simulink model "HEV_Simu_V1_1_SfuncPtbs"  (R2018b)
settings: configuration reference "Config_Plant" (kept outside this file)
PreLoadFcn:
  | HevSimuVccWs_V1_PreLoad
  | %プラントモデルのコールバック・プリロード関数のバス定義
  | Driver_PreLoad
  | HEVPlant_Ptbs_V1_BusInfo
  | CtrlStrct_SmplCAN_BusInfo
StartFcn:
  | tic
StopFcn:
  | toc
  | disp(['実時間の' num2str(max(tout)/toc) '倍速'])
libraries: CAN_Lib_V1 x4, simulink x2
settings Model: Creator=E00026  LastModifiedBy=E00026
settings ConfigSetRef: SourceLocation=Base Workspace

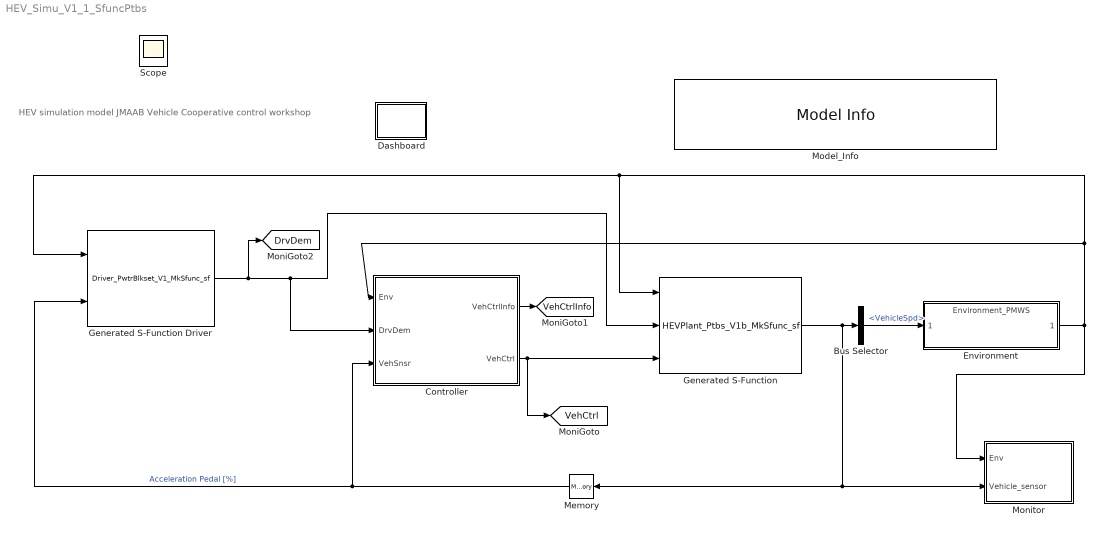
== system HEV_Simu_V1_1_SfuncPtbs ==
  note: HEV simulation model
      | JMAAB Vehicle Cooperative control workshop
  Bus Selector : BusSelector  OutputSignals=Brake_sensor.VehicleSpd
  Controller : Subsystem  TreatAsAtomicUnit=on  VariantControl=VarObj_CtrlStruct_CAN_VNT_Level_2
  Dashboard : Subsystem
  Environment : ModelReference  ModelNameDialog=Environment_PMWS.slx  SimulationMode=Normal  ModelReferenceVersion=1.1287
  Generated S-Function : S-Function  FunctionName=HEVPlant_Ptbs_V1b_MkSfunc_sf  Parameters=sfcnParam1, sfcnParam2, sfcnParam3, sfcnParam4, sfcnParam5, sfcnParam6, sfcnParam7, sfcnParam8, sfcnParam9, sfcnParam10, sfcnParam11, sfcnParam12, sfcnParam13, sfcnParam14, sfcnParam15, sfcnParam16, sfcnParam17, sfcnParam18, sfcnParam19, sfcnParam20, sfcnParam21, sfcnParam22, sfcnParam23, sfcnParam24, sfcnParam25, sfcnParam26, sfcnParam27, sfcnParam28, sfcnParam29, sfcnParam30, sfcnParam31, sfcnParam32, sfcnParam33, sfcnParam34, sfcnParam35, sfcnParam36, sfcnParam37, sfcnParam38, sfcnParam39, sfcnParam40, sfcnParam41, sfcnParam42, sfcnParam43, sfcnParam44, sfcnParam45, sfcnParam46, sfcnParam47, sfcnParam48, sfcnParam49, sfcnParam50, sfcnParam51, sfcnParam52, sfcnParam53, sfcnParam54, sfcnParam55, sfcnParam56, sfcnParam57, sfcnParam58, sfcnParam59, sfcnParam60, sfcnParam61, sfcnParam62, sfcnParam63, sfcnParam64, sfcnParam65, sfcnParam66, sfcnParam67, sfcnParam68, sfcnParam69, sfcnParam70, sfcnParam71, sfcnParam72, sfcnParam73, sfcnParam74, sfcnParam75, sfcnParam76, sfcnParam77, sfcnParam78, sfcnParam79, sfcnParam80, sfcnParam81, sfcnParam82, sfcnParam83, sfcnParam84, sfcnParam85, sfcnParam86, sfcnParam87, sfcnParam88, sfcnParam89, sfcnParam90, sfcnParam91, sfcnParam92, sfcnParam93, sfcnParam94, sfcnParam95, sfcnParam96, sfcnParam97, sfcnParam98, sfcnParam99, sfcnParam100, sfcnParam101, sfcnParam102, sfcnParam103, sfcnParam104, sfcnParam105, sfcnParam106, sfcnParam107, sfcnParam108, sfcnParam109, sfcnParam110, sfcnParam111, sfcnParam112, sfcnParam113, sfcnParam114, sfcnParam115, sfcnParam116, sfcnParam117, sfcnParam118, sfcnParam119, sfcnParam120, sfcnParam121, sfcnParam122, sfcnParam123  SFunctionModules=""  SFunctionDeploymentMode=off  EnableBusSupport=off  mask{rtw_sf_name=HEVPlant_Ptbs_V1b_MkSfunc_sf, showVar=off, sfcnParam1=[3.421], sfcnParam2=[1.0], sfcnParam3=[0.3], sfcnParam4=[10.0], sfcnParam5=[10.0], sfcnParam6=[5000.0], sfcnParam7=[1000.0], sfcnParam8=[0.1], sfcnParam9=[2.27], sfcnParam10=[4.2], sfcnParam11=[7.0], sfcnParam12=[243.1, 253.1, 263.1, 273.1, 283.1, 298.1, 313.1], sfcnParam13=[0.0, 0.01, 0.02, 0.03, 0.04, 0.05, 0.06, 0.07, 0.08, 0.09, 0.1, 0.11, 0.12, 0.13, 0.14, 0.15, 0.16, 0.17, 0.18, 0.19, 0.2, 0.21, 0.22, 0.23, 0.24, 0.25, 0.26, 0.27, 0.28, 0.29, 0.3, 0.31, 0.32, 0.33, 0.34, 0.35, 0.36, 0.37, 0.38, 0.39, 0.4, 0.41, 0.42, 0.43, 0.44, 0.45, 0.46, 0.47, 0.48, 0.49, 0.5, 0.51, 0.52, 0.53, 0.54, 0.55, 0.56, 0.57, 0.58, 0.59, 0.6, 0.61, 0.62, 0.63, 0.64, 0.65, 0.66, 0.67, 0.68, 0.69, 0.7, 0.71, 0.72, 0.73, 0.74, 0.75, 0.76, 0.77, 0.78, 0.79, 0.8, 0.81, 0.82, 0.83, 0.84, 0.85, 0.86, 0.87, 0.88, 0.89, 0.9, 0.91, 0.92, 0.93, 0.94, 0.95, 0.96, 0.97, 0.98, 0.99, 1.0], sfcnParam14=[0.0, 0.2, 0.4, 0.6, 0.8, 1.0], sfcnParam15=[0.29], sfcnParam16=[2.8, 3.228, 3.284, 3.361, 3.408, 3.427, 3.472, 3.477, 3.493, 3.504, 3.516, 3.528, 3.537, 3.545, 3.555, 3.561, 3.566, 3.576, 3.587, 3.589, 3.594, 3.6, 3.608, 3.61, 3.616, 3.619, 3.626, 3.632, 3.637, 3.64, 3.645, 3.646, 3.652, 3.655, 3.658, 3.661, 3.664, 3.668, 3.673, 3.678, 3.68, 3.681, 3.686, 3.692, 3.699, 3.702, 3.705, 3.71, 3.717, 3.723, 3.728, 3.733, 3.735, 3.742, 3.749, 3.755, 3.761, 3.768, 3.773, 3.78, 3.791, 3.798, 3.798, 3.814, 3.818, 3.825, 3.841, 3.846, 3.855, 3.863, 3.877, 3.885, 3.894, 3.907, 3.919, 3.926, 3.935, 3.944, 3.954, 3.964, 3.974, 3.988, 3.998, 4.014, 4.029, 4.034, 4.047, 4.065, 4.074, 4.086, 4.097, 4.131, 4.126, 4.138, 4.15, 4.18, 4.174, 4.187, 4.207, 4.231, 4.221], sfcnParam17=[4000.0], sfcnParam18=[4000.0], sfcnParam19=[10000.0], sfcnParam20=[10000.0], sfcnParam21=[0.0], sfcnParam22=[0.0], sfcnParam23=[-1.0, 0.0, 1.0, 2.0, 3.0, 4.0, 5.0], sfcnParam24=[0.0], sfcnParam25=[0.8], sfcnParam26=[0.8], sfcnParam27=[0.025], sfcnParam28=[0.3], sfcnParam29=[0.128, 0.01, 0.128, 0.1, 0.062, 0.028, 0.01], sfcnParam30=[0.01], sfcnParam31=[0.01], sfcnParam32=[5000.0], sfcnParam33=[0.15], sfcnParam34=[0.15], sfcnParam35=[-4.47, 1.0, 4.47, 2.47, 1.47, 1.0, 0.8], sfcnParam36=[2.0], sfcnParam37=[220000.0], sfcnParam38=[220000.0], sfcnParam39=[2.0], sfcnParam40=[1.0], sfcnParam41=[76.19047619047619], sfcnParam42=[101325.0], sfcnParam43=[0.007], sfcnParam44=[0.007], sfcnParam45=[0.0], sfcnParam46=[0.0], sfcnParam47=[0.0015], sfcnParam48=[0.0015], sfcnParam49=[8.5E-5], sfcnParam50=[8.5E-5], sfcnParam51=[0.0], sfcnParam52=[0.0], sfcnParam53=[0.0], sfcnParam54=[0.0], sfcnParam55=[0.9], sfcnParam56=[0.9], sfcnParam57=[-0.4], sfcnParam58=[-0.4], sfcnParam59=[0.2], sfcnParam60=reshape([0.008846, 0.006389, 0.004364, 0.002031, 0.001443, 0.0005603, 0.001028, 0.009319, 0.006554, 0.004101, 0.002563, 0.001825, 0.0007192, 0.001338, 0.009027, 0.005553, 0.00406, 0.002532, 0.001795, 0.0006887, 0.001, 0.00847, 0.005525, 0.003452, 0.00246, 0.001778, 0.0007557, 0.001536, 0.01032, 0.006043, 0.003846, 0.002716, 0.001924, 0.0007355, 0.001546, 0.01314, 0.007805, 0.004517, 0.003047, 0.002234, 0.001014, 0.002789], 7, 6), sfcnParam61=[0.0], sfcnParam62=[0.0], sfcnParam63=[0.1778], sfcnParam64=[0.1778], sfcnParam65=[273.0], sfcnParam66=[0.02], sfcnParam67=[0.4], sfcnParam68=[0.4], sfcnParam69=[2.0], sfcnParam70=[2.0], sfcnParam71=[1.56], sfcnParam72=[1.22], sfcnParam73=[0.001], sfcnParam74=[0.03], sfcnParam75=[0.003, 0.001, 0.003, 0.0025, 0.002, 0.001, 0.001], sfcnParam76=[0.001], sfcnParam77=[0.001], sfcnParam78=[0.001], sfcnParam79=[0.001], sfcnParam80=[1.0], sfcnParam81=[0.05], sfcnParam82=[0.05], sfcnParam83=[0.0], sfcnParam84=[0.0], sfcnParam85=[0.9, 0.9, 0.9, 0.9, 0.9, 0.95, 0.95], sfcnParam86=reshape([-13.1081458684774, 4.32139921766168, 20.757244711379, 35.9627269414642, 49.8552657259726, 62.5657141177372, 74.477004401576, 86.1003984024147, 97.7334079817966, 109.479762957418, 121.326441846396, 133.101497884419, 144.820899208063, 156.736480114968, 169.114710642361, 182.092709016827, 195.59958423146, 209.368412323981, 223.02848004595, 236.207526223604, -14.1627478704748, 3.99894401639278, 21.2867510394, 37.4521026772137, 52.3565546365145, 66.079624495863, 79.0243307343782, 91.7565682685391, 104.540141180755, 117.253813854056, 129.726304313329, 141.881214846407, 153.93087450367, 166.194306611943, 178.940714413665, 192.3215915833, 206.228422981382, 220.31244451237, 234.137078836663, 247.312038629797, -15.7784609520012, 2.89292159663557, 20.7363542505055, 37.502335524464, 53.0509548864367, 67.5025986362754, 81.3135932041197, 95.0325125167302, 108.810465740463, 122.355917599999, 135.439918107165, 148.199351304314, 160.955784626292, 173.836234315838, 187.087035458638, 200.927324396312, 215.214502850912, 229.514564126309, 243.353035073859, 256.366094046404, -17.42253942172, 1.64416808773342, 19.8409346288691, 36.9233984519825, 52.8290032980595, 67.7977424348511, 82.3245510739081, 96.8466026217949, 111.383077007938, 125.653415687543, 139.51810242633, 153.176047542526, 166.789387360173, 180.265364531531, 193.934331712532, 208.094949306354, 222.553115988777, 236.807747408065, 250.406930317565, 263.064113811605, -18.9093330140012, 0.468673396230884, 18.909574147504, 36.1995377541326, 52.3840426102553, 67.8062848977726, 82.9383422780821, 98.068344684537, 113.145959398055, 128.053904824993, 142.823295869735, 157.475130990134, 171.799449524305, 185.674025487578, 199.53883414199, 213.697313618018, 227.940691948826, 241.792900146554, 254.902489131827, 267.076281290808, -20.3238171022812, -0.775207212324744, 17.8042755322396, 35.2637545810877, 51.7007503585347, 67.4992335531143, 83.0841953272912, 98.6206039616237, 114.008086889125, 129.279732299868, 144.630713577572, 159.966846530691, 174.869524788418, 189.128197558793, 203.056423425079, 216.938114500504, 230.662578894656, 243.917825141355, 256.489704414577, 268.231292584403, -21.7238586333832, -2.10073707536401, 16.5254772659256, 34.0668553207516, 50.6513840229173, 66.6631193971417, 82.4787130004125, 98.1766276641439, 113.598772867598, 128.82687247386, 144.167755344636, 159.567031205502, 174.649500781715, 189.180343691042, 203.252566971657, 216.975565766582, 230.297947352186, 243.112061758629, 255.331922415077, 266.799887767717, -23.1529035628035, -3.50862107436012, 15.0855958673793, 32.6058441274955, 49.2251524655886, 65.3151203705212, 81.1933702605176, 96.8521721846929, 112.043378968826, 126.808816875754, 141.565819466444, 156.460712503163, 171.383162564817, 186.232253968382, 200.785359211282, 214.707679019995, 227.888303712579, 240.423272401809, 252.341328875323, 263.495565903738, -24.6884602505442, -5.06028470965873, 13.4498911250713, 30.8989322512799, 47.5134968647191, 63.6435466094273, 79.5336209695535, 95.087170410946, 109.948780519903, 124.055675651399, 137.939311973562, 152.1103125245, 166.849299169569, 182.224256255854, 197.494951561167, 211.705705526533, 224.705940883011, 236.845866634963, 248.276832730234, 258.916438206755, -26.362684645267, -6.71203349342875, 11.7522265884483, 29.1624870834213, 45.7908651096087, 61.9616994275867, 77.8492465663741, 93.3376125442893, 108.050693576822, 121.779776759549, 134.991731787931, 148.557791123037, 163.149781208938, 178.807064638401, 194.343816615511, 208.400898889072, 220.908829093315, 232.436458175814, 243.265245628093, 253.353482786698, -28.1859502990691, -8.38741975881464, 10.1532754693627, 27.6329419979166, 44.3421988978963, 60.5787546917719, 76.4821091386121, 91.9935854422957, 106.822280331792, 120.653676977018, 133.763700644443, 147.149800719098, 161.62761641339, 176.981869454773, 191.902393007376, 205.207199013255, 216.948288417291, 227.717031148394, 237.842323295526, 247.316194797038, -30.2417219781918, -10.1224652436348, ...(+3220 chars)), sfcnParam87=[0.0, 2.63157894736842, 5.26315789473684, 7.89473684210526, 10.5263157894737, 13.1578947368421, 15.7894736842105, 18.4210526315789, 21.0526315789474, 23.6842105263158, 26.3157894736842, 28.9473684210526, 31.5789473684211, 34.2105263157895, 36.8421052631579, 39.4736842105263, 42.1052631578947, 44.7368421052632, 47.3684210526316, 50.0], sfcnParam88=[1000.0, 1302.63157894737, 1605.26315789474, 1907.89473684211, 2210.52631578947, 2513.15789473684, 2815.78947368421, 3118.42105263158, 3421.05263157895, 3723.68421052632, 4026.31578947368, 4328.94736842105, 4631.57894736842, 4934.21052631579, 5236.84210526316, 5539.47368421053, 5842.1052631579, 6144.73684210526, 6447.36842105263, 6750.0], sfcnParam89=[9.81], sfcnParam90=[0.0], sfcnParam91=[0.0], sfcnParam92=[0.5], sfcnParam93=[10.0], sfcnParam94=[10.0], sfcnParam95=[1.0], sfcnParam96=[1.0], sfcnParam97=[1.0], sfcnParam98=[1.0], sfcnParam99=[1723.2], sfcnParam100=[0.2], sfcnParam101=[0.2], sfcnParam102=[0.3], sfcnParam103=[0.3], sfcnParam104=[0.4], sfcnParam105=[0.6], sfcnParam106=[2.0], sfcnParam107=[2.0], sfcnParam108=[0.0], sfcnParam109=[0.0], sfcnParam110=[0.0], sfcnParam111=[0.0], sfcnParam112=[0.0], sfcnParam113=[0.0], sfcnParam114=[124000.0], sfcnParam115=[220000.0], sfcnParam116=[220000.0], sfcnParam117=[0.02], sfcnParam118=[0.0], sfcnParam119=[0.0], sfcnParam120=[1.0E-6], sfcnParam121=[307.0], sfcnParam122=[0.15], sfcnParam123=[0.0]}
      mask prompts: rtw_sf_name "Simulink:masks:GenSFuncName_MP"; showVar "Simulink:masks:GenSFuncShowModuleList_MP"; sfcnParam1 "DiffRatio:"; sfcnParam2 "MotGbRatio:"; sfcnParam3 "RWheel:"; sfcnParam4 "b_axle:"; sfcnParam5 "b_driveshaft:"; sfcnParam6 "k_axle:"; sfcnParam7 "k_driveshaft:"; sfcnParam8 "wc_shaft:"; sfcnParam9 "VehicleBody1DOFLongitudinal_Af:"; sfcnParam10 "LithiumIonBatteryPack_BattCapIn:"; sfcnParam11 "LithiumIonBatteryPack_BattCharg:"; sfcnParam12 "LithiumIonBatteryPack_BattTempB:"; sfcnParam13 "LithiumIonBatteryPack_CapLUTBp:"; sfcnParam14 "LithiumIonBatteryPack_CapSOCBp:"; sfcnParam15 "VehicleBody1DOFLongitudinal_Cd:"; sfcnParam16 "LithiumIonBatteryPack_Em:"; sfcnParam17 "LongitudinalWheelFront_FNOMIN:"; sfcnParam18 "LongitudinalWheelRear_FNOMIN:"; sfcnParam19 "LongitudinalWheelFront_FZMAX:"; sfcnParam20 "LongitudinalWheelRear_FZMAX:"; sfcnParam21 "LongitudinalWheelFront_FZMIN:"; sfcnParam22 "LongitudinalWheelRear_FZMIN:"; sfcnParam23 "AutomatedManualTransmission_G:"; sfcnParam24 "AutomatedManualTransmission_G_o:"; sfcnParam25 "LongitudinalWheelFront_Iyy:"; sfcnParam26 "LongitudinalWheelRear_Iyy:"; sfcnParam27 "OpenDifferential_Jd:"; sfcnParam28 "AutomatedManualTransmission_Jin:"; sfcnParam29 "AutomatedManualTransmission_Jou:"; sfcnParam30 "OpenDifferential_Jw1:"; sfcnParam31 "OpenDifferential_Jw2:"; sfcnParam32 "AutomatedManualTransmission_K_c:"; sfcnParam33 "LongitudinalWheelFront_Lrel:"; sfcnParam34 "LongitudinalWheelRear_Lrel:"; sfcnParam35 "AutomatedManualTransmission_N:"; sfcnParam36 "VehicleBody1DOFLongitudinal_NF:"; sfcnParam37 "LongitudinalWheelFront_NOMPRES:"; sfcnParam38 "LongitudinalWheelRear_NOMPRES:"; sfcnParam39 "VehicleBody1DOFLongitudinal_NR:"; sfcnParam40 "LithiumIonBatteryPack_Np:"; sfcnParam41 "LithiumIonBatteryPack_Ns:"; sfcnParam42 "VehicleBody1DOFLongitudinal_Pab:"; sfcnParam43 "LongitudinalWheelFront_QSY1:"; sfcnParam44 "LongitudinalWheelRear_QSY1:"; sfcnParam45 "LongitudinalWheelFront_QSY2:"; sfcnParam46 "LongitudinalWheelRear_QSY2:"; sfcnParam47 "LongitudinalWheelFront_QSY3:"; sfcnParam48 "LongitudinalWheelRear_QSY3:"; sfcnParam49 "LongitudinalWheelFront_QSY4:"; sfcnParam50 "LongitudinalWheelRear_QSY4:"; sfcnParam51 "LongitudinalWheelFront_QSY5:"; sfcnParam52 "LongitudinalWheelRear_QSY5:"; sfcnParam53 "LongitudinalWheelFront_QSY6:"; sfcnParam54 "LongitudinalWheelRear_QSY6:"; sfcnParam55 "LongitudinalWheelFront_QSY7:"; sfcnParam56 "LongitudinalWheelRear_QSY7:"; sfcnParam57 "LongitudinalWheelFront_QSY8:"; sfcnParam58 "LongitudinalWheelRear_QSY8:"; sfcnParam59 "AutomatedManualTransmission_R:"; sfcnParam60 "LithiumIonBatteryPack_RInt:"; sfcnParam61 "HardPointCoordinateTransformFro:"; sfcnParam62 "HardPointCoordinateTransformRea:"; sfcnParam63 "LongitudinalWheelFront_Rm:"; sfcnParam64 "LongitudinalWheelRear_Rm:"; sfcnParam65 "VehicleBody1DOFLongitudinal_T:"; sfcnParam66 "MappedMotor_Tc:"; sfcnParam67 "LongitudinalWheelFront_UNLOADED:"; sfcnParam68 "LongitudinalWheelRear_UNLOADED_:"; sfcnParam69 "LongitudinalWheelFront_VXLOW:"; sfcnParam70 "LongitudinalWheelRear_VXLOW:"; sfcnParam71 "VehicleBody1DOFLongitudinal_a:"; sfcnParam72 "VehicleBody1DOFLongitudinal_b:"; sfcnParam73 "OpenDifferential_bd:"; sfcnParam74 "AutomatedManualTransmission_bin:"; sfcnParam75 "AutomatedManualTransmission_bou:"; sfcnParam76 "LongitudinalWheelFront_br:"; sfcnParam77 "LongitudinalWheelRear_br:"; sfcnParam78 "OpenDifferential_bw1:"; sfcnParam79 "OpenDifferential_bw2:"; sfcnParam80 "CompareToConstant_const:"; sfcnParam81 "LongitudinalWheelFront_disk_abo:"; sfcnParam82 "LongitudinalWheelRear_disk_abor:"; sfcnParam83 "DriveshaftCompliance_domega_o:"; sfcnParam84 "AxleCompliance_domega_o:"; sfcnParam85 "AutomatedManualTransmission_eta:"; sfcnParam86 "MappedCIEngine_f_tbrake:"; sfcnParam87 "MappedCIEngine_f_tbrake_f_bpt:"; sfcnParam88 "MappedCIEngine_f_tbrake_n_bpt:"; sfcnParam89 "VehicleBody1DOFLongitudinal_g:"; sfcnParam90 "LongitudinalWheelFront_gamma:"; sfcnParam91 "LongitudinalWheelRear_gamma:"; sfcnParam92 "VehicleBody1DOFLongitudinal_h:"; sfcnParam93 "LongitudinalWheelFront_kappamax:"; sfcnParam94 "LongitudinalWheelRear_kappamax:"; sfcnParam95 "LongitudinalWheelFront_lam_My:"; sfcnParam96 "LongitudinalWheelRear_lam_My:"; sfcnParam97 "LongitudinalWheelFront_lam_x:"; sfcnParam98 "LongitudinalWheelRear_lam_x:"; sfcnParam99 "VehicleBody1DOFLongitudinal_m:"; sfcnParam100 "LongitudinalWheelFront_mu_kinet:"; sfcnParam101 "LongitudinalWheelRear_mu_kineti:"; sfcnParam102 "LongitudinalWheelFront_mu_stati:"; sfcnParam103 "LongitudinalWheelRear_mu_static:"; sfcnParam104 "AutomatedManualTransmission_muk:"; sfcnParam105 "AutomatedManualTransmission_mus:"; sfcnParam106 "LongitudinalWheelFront_num_pads:"; sfcnParam107 "LongitudinalWheelRear_num_pads:"; sfcnParam108 "AutomatedManualTransmission_ome:"; sfcnParam109 "LongitudinalWheelFront_omegao:"; sfcnParam110 "LongitudinalWheelRear_omegao:"; sfcnParam111 "AutomatedManualTransmission_o_f:"; sfcnParam112 "OpenDifferential_omegaw1o:"; sfcnParam113 "OpenDifferential_omegaw2o:"; sfcnParam114 "MappedMotor_power_max:"; sfcnParam115 "LongitudinalWheelFront_press:"; sfcnParam116 "LongitudinalWheelRear_press:"; sfcnParam117 "AutomatedManualTransmission_tau:"; sfcnParam118 "DriveshaftCompliance_theta_o:"; sfcnParam119 "AxleCompliance_theta_o:"; sfcnParam120 "div0protectabspoly1_thresh:"; sfcnParam121 "MappedMotor_torque_max:"; sfcnParam122 "AutomatedManualTransmission_ts:"; sfcnParam123 "VehicleBody1DOFLongitudinal_xdo:"
      mask help: Simulink:masks:GenSFuncDesc_MD
      mask init:
      | displist = '';
      | if ~strcmp(get_param(gcb, 'FunctionName'), rtw_sf_name);
      |   set_param(gcb, 'FunctionName', rtw_sf_name);
      | end
      | % Check if we are generating code
      | rtw_mode = false;
      | if strcmpi(get_param(bdroot(gcb),'SimulationStatus'),'Initializing')
      | 	rtw_mode = strcmpi(get_param(bdroot(gcb),'BuildingRTWCode'),'on') && ...
      | 		~strcmpi(get_param(bdroot(gcb),'TargetStyle'),'SimulationTarget');
      | end
      | if showVar || rtw_mode
      | 	if exist('rtwsfunc') == 2 | exist('rtwsfunc') == 6
      | 		tmplist = rtwsfunc(rtw_sf_name,gcb);
      | 		tmplist = DAStudio.message('Simulink:masks:GenSFuncListOfModules_IC', tmplist);
      | 	elseif showVar
      | 		tmplist1 = DAStudio.message('Simulink:masks:GenSFuncListOfModules_IC', '');
      |         tmplist2 = DAStudio.message('Simulink:masks:GenSFuncNotLicensed_IC');
      |         tmplist = [tmplist1 tmplist2];
      |  	end
      | end
      | if showVar
      |   displist = tmplist;
      | end
      settings: CopyFcn=|
      | if ~strcmp(get_param(gcb,'Linkstatus'),'none') && ...
      | ~strcmp(get_param(gcb,'Linkstatus'),'implicit')
      |   set_param(gcb,'LinkStatus','none');
      | end
      mask Help: eval('feval(''rtwprivate'',''rtwhelpview'',''rtw_sfcn_block'')');
      mask Display:
      | port_label('input',1,'Env');
      | port_label('input',2,'DrvDem');
      | port_label('input',3,'Controller');
      | port_label('output',1,'Vehicle_sensor');
  Generated S-Function Driver : S-Function  FunctionName=Driver_PwtrBlkset_V1_MkSfunc_sf  Parameters=sfcnParam1, sfcnParam2, sfcnParam3, sfcnParam4, sfcnParam5, sfcnParam6, sfcnParam7  SFunctionModules=""  SFunctionDeploymentMode=off  EnableBusSupport=off  SFcnStateName=DWORK0  mask{rtw_sf_name=Driver_PwtrBlkset_V1_MkSfunc_sf, showVar=off, sfcnParam1=[1.0], sfcnParam2=[0.1], sfcnParam3=[0.0], sfcnParam4=[0.2], sfcnParam5=[1.0], sfcnParam6=[0.01], sfcnParam7=[5.0]}
      mask prompts: rtw_sf_name "Simulink:masks:GenSFuncName_MP"; showVar "Simulink:masks:GenSFuncShowModuleList_MP"; sfcnParam1 "LongitudinalDriverModel1_Kaw:"; sfcnParam2 "LongitudinalDriverModel1_Kff:"; sfcnParam3 "LongitudinalDriverModel1_Kg:"; sfcnParam4 "LongitudinalDriverModel1_Ki:"; sfcnParam5 "LongitudinalDriverModel1_Kp:"; sfcnParam6 "LongitudinalDriverModel1_tauerr:"; sfcnParam7 "LongitudinalDriverModel1_vnom:"
      mask help: Simulink:masks:GenSFuncDesc_MD
      mask init: same as HEV_Simu_V1_1_SfuncPtbs/Generated S-Function
      settings: SFcnIsStateOwnerBlock=on
      settings: CopyFcn=|
      | if ~strcmp(get_param(gcb,'Linkstatus'),'none') && ...
      | ~strcmp(get_param(gcb,'Linkstatus'),'implicit')
      |   set_param(gcb,'LinkStatus','none');
      | end
      mask Help: eval('feval(''rtwprivate'',''rtwhelpview'',''rtw_sfcn_block'')');
      mask Display:
      | port_label('input',1,'Env');
      | port_label('input',2,'Vehicle_sensor');
      | port_label('output',1,'DrvDem');
  Memory : Memory
  Model_Info : simulink/Model-Wide Utilities/Model Info  Frame=on  DisplayStringWithTags=|  HorizontalTextAlignment=Left  LeftAlignmentValue=0.02
      | Version  %<ModelVersion>
      | LastModifided by %<LastModifiedBy>  Date %<LastModificationDate>
      | Description  %<Description>
  Monitor : Subsystem
  Scope : Scope
  tag scope: DrvDem=global, VehCtrl=global, VehCtrlInfo=global
  wires:
  Environment/1 -> Controller/1(Env), Generated S-Function/1, Generated S-Function Driver/1, Monitor/1(Env)
  Controller/1(VehCtrlInfo) -> [VehCtrlInfo]
  Generated S-Function/1 -> Monitor/2(Vehicle_sensor), Memory/1, Bus Selector/1
  Generated S-Function Driver/1 -> [DrvDem], Controller/2(DrvDem), Generated S-Function/2
  Memory/1 -> Controller/3(VehSnsr), Generated S-Function Driver/2  "Acceleration Pedal [%]"
  Controller/2(VehCtrl) -> Generated S-Function/3, [VehCtrl]
  Bus Selector/1 -> Environment/1  "<VehicleSpd>"

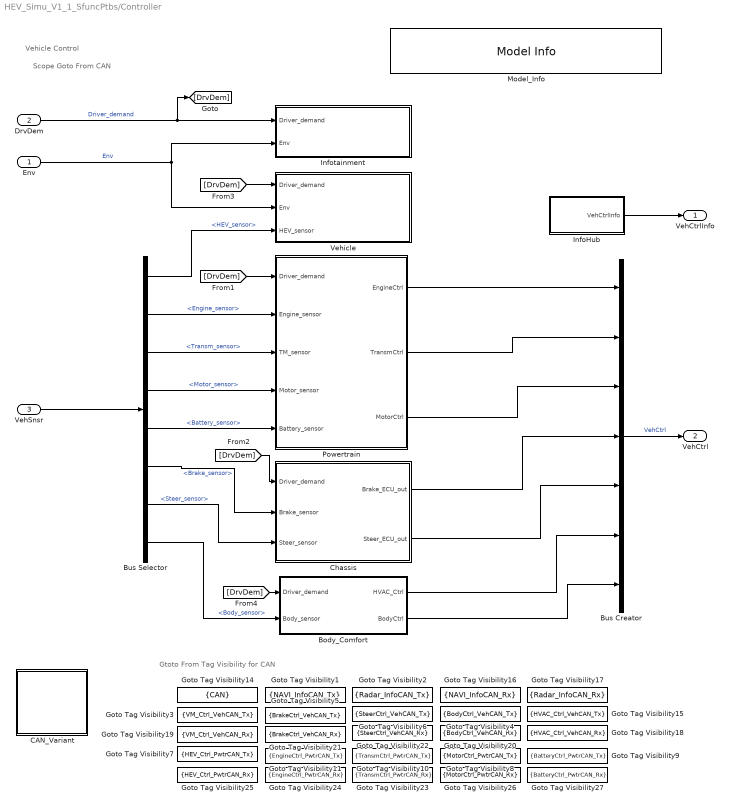
== system HEV_Simu_V1_1_SfuncPtbs/Controller ==
  note: Scope Goto From CAN
  note: Gtoto From Tag Visibility for CAN
  note: Vehicle Control
  Env : Inport  OutDataTypeStr=Bus: Environment_Bus
      settings: AttributesFormatString=<%<OutDataTypeStr>>
  DrvDem : Inport  Port=2  OutDataTypeStr=Bus: Driver_demand_Bus
      settings: AttributesFormatString=%<OutDataTypeStr>
  VehSnsr : Inport  Port=3  OutDataTypeStr=Bus: Vehicle_sensor_Bus
      settings: AttributesFormatString=<%<OutDataTypeStr>>
  Body_Comfort : Subsystem
  Bus Creator : BusCreator  Inputs=7  OutDataTypeStr=Bus: Ctrl_intg_Bus
      settings: AttributesFormatString=%<OutDataTypeStr>
  Bus Selector : BusSelector  OutputSignals=HEV_sensor,Engine_sensor,Transm_sensor,Motor_sensor,Battery_sensor,Brake_sensor,Steer_sensor,Body_sensor
  CAN_Variant : Subsystem  Variant=on
  Chassis : Subsystem
  Goto Tag Visibility1 : GotoTagVisibility  GotoTag=NAVI_InfoCAN_Tx
  Goto Tag Visibility10 : GotoTagVisibility  GotoTag=TransmCtrl_PwtrCAN_Tx
  Goto Tag Visibility11 : GotoTagVisibility  GotoTag=EngineCtrl_PwtrCAN_Tx
  Goto Tag Visibility14 : GotoTagVisibility  GotoTag=CAN
  Goto Tag Visibility15 : GotoTagVisibility  GotoTag=HVAC_Ctrl_VehCAN_Tx
  Goto Tag Visibility16 : GotoTagVisibility  GotoTag=NAVI_InfoCAN_Rx
  Goto Tag Visibility17 : GotoTagVisibility  GotoTag=Radar_InfoCAN_Rx
  Goto Tag Visibility18 : GotoTagVisibility  GotoTag=HVAC_Ctrl_VehCAN_Rx
  Goto Tag Visibility19 : GotoTagVisibility  GotoTag=VM_Ctrl_VehCAN_Rx
  Goto Tag Visibility2 : GotoTagVisibility  GotoTag=Radar_InfoCAN_Tx
  Goto Tag Visibility20 : GotoTagVisibility  GotoTag=BodyCtrl_VehCAN_Rx
  Goto Tag Visibility21 : GotoTagVisibility  GotoTag=BrakeCtrl_VehCAN_Rx
  Goto Tag Visibility22 : GotoTagVisibility  GotoTag=SteerCtrl_VehCAN_Rx
  Goto Tag Visibility23 : GotoTagVisibility  GotoTag=TransmCtrl_PwtrCAN_Rx
  Goto Tag Visibility24 : GotoTagVisibility  GotoTag=EngineCtrl_PwtrCAN_Rx
  Goto Tag Visibility25 : GotoTagVisibility  GotoTag=HEV_Ctrl_PwtrCAN_Rx
  Goto Tag Visibility26 : GotoTagVisibility  GotoTag=MotorCtrl_PwtrCAN_Rx
  Goto Tag Visibility27 : GotoTagVisibility  GotoTag=BatteryCtrl_PwtrCAN_Rx
  Goto Tag Visibility3 : GotoTagVisibility  GotoTag=VM_Ctrl_VehCAN_Tx
  Goto Tag Visibility4 : GotoTagVisibility  GotoTag=BodyCtrl_VehCAN_Tx
  Goto Tag Visibility5 : GotoTagVisibility  GotoTag=BrakeCtrl_VehCAN_Tx
  Goto Tag Visibility6 : GotoTagVisibility  GotoTag=SteerCtrl_VehCAN_Tx
  Goto Tag Visibility7 : GotoTagVisibility  GotoTag=HEV_Ctrl_PwtrCAN_Tx
  Goto Tag Visibility8 : GotoTagVisibility  GotoTag=MotorCtrl_PwtrCAN_Tx
  Goto Tag Visibility9 : GotoTagVisibility  GotoTag=BatteryCtrl_PwtrCAN_Tx
  InfoHub : Subsystem
  Infotainment : Subsystem
  Model_Info : simulink/Model-Wide Utilities/Model Info  Frame=on  DisplayStringWithTags=|  HorizontalTextAlignment=Left  LeftAlignmentValue=0.02
      | Version  %<ModelVersion>
      | LastModifided by %<LastModifiedBy>  Date %<LastModificationDate>
      | Description  %<Description>
  Powertrain : Subsystem
  Vehicle : Subsystem
  VehCtrlInfo : Outport  OutDataTypeStr=Bus: IntgCtrl_Info_Bus
      settings: AttributesFormatString=<%<OutDataTypeStr>>
  VehCtrl : Outport  Port=2  OutDataTypeStr=Bus: Ctrl_intg_Bus
      settings: AttributesFormatString=<%<OutDataTypeStr>>
  wires:
  DrvDem/1 -> [DrvDem], Infotainment/1(Driver_demand)  "Driver_demand"
  [DrvDem] -> Powertrain/1(Driver_demand)
  Chassis/1(Brake_ECU_out) -> Bus Creator/4
  Bus Selector/5 -> Powertrain/5(Battery_sensor)  "<Battery_sensor>"
  [DrvDem] -> Vehicle/1(Driver_demand)
  Bus Creator/1 -> VehCtrl/1  "VehCtrl"
  Body_Comfort/1(HVAC_Ctrl) -> Bus Creator/6
  Powertrain/1(EngineCtrl) -> Bus Creator/1
  Bus Selector/1 -> Vehicle/3(HEV_sensor)  "<HEV_sensor>"
  Bus Selector/8 -> Body_Comfort/2(Body_sensor)  "<Body_sensor>"
  Bus Selector/4 -> Powertrain/4(Motor_sensor)  "<Motor_sensor>"
  [DrvDem] -> Body_Comfort/1(Driver_demand)
  VehSnsr/1 -> Bus Selector/1
  Body_Comfort/2(BodyCtrl) -> Bus Creator/7
  Bus Selector/7 -> Chassis/3(Steer_sensor)  "<Steer_sensor>"
  Bus Selector/2 -> Powertrain/2(Engine_sensor)  "<Engine_sensor>"
  [DrvDem] -> Chassis/1(Driver_demand)
  Bus Selector/6 -> Chassis/2(Brake_sensor)  "<Brake_sensor>"
  Powertrain/2(TransmCtrl) -> Bus Creator/2
  InfoHub/1(VehCtrlInfo) -> VehCtrlInfo/1
  Bus Selector/3 -> Powertrain/3(TM_sensor)  "<Transm_sensor>"
  Env/1 -> Vehicle/2(Env), Infotainment/2(Env)  "Env"
  Powertrain/3(MotorCtrl) -> Bus Creator/3
  Chassis/2(Steer_ECU_out) -> Bus Creator/5

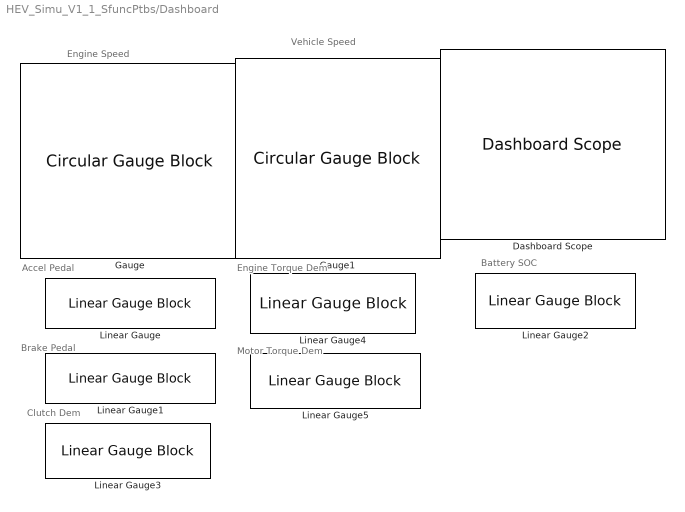
== system HEV_Simu_V1_1_SfuncPtbs/Dashboard ==
  note: Battery SOC
  note: Brake Pedal
  note: Accel Pedal
  note: Engine Speed
  note: Vehicle Speed
  note: Engine Torque Dem
  note: Clutch Dem
  note: Motor Torque Dem
  Dashboard Scope : DashboardScope  TimeSpan=30  Ymin=0  Ymax=30
  Gauge : CircularGaugeBlock  ScaleMax=4000
  Gauge1 : CircularGaugeBlock  ScaleMax=160  TickInterval=20
  Linear Gauge{,1..2,4} (4 alike) : LinearGaugeBlock
  Linear Gauge3 : LinearGaugeBlock  ScaleMax=1
  Linear Gauge5 : LinearGaugeBlock  ScaleMin=-100

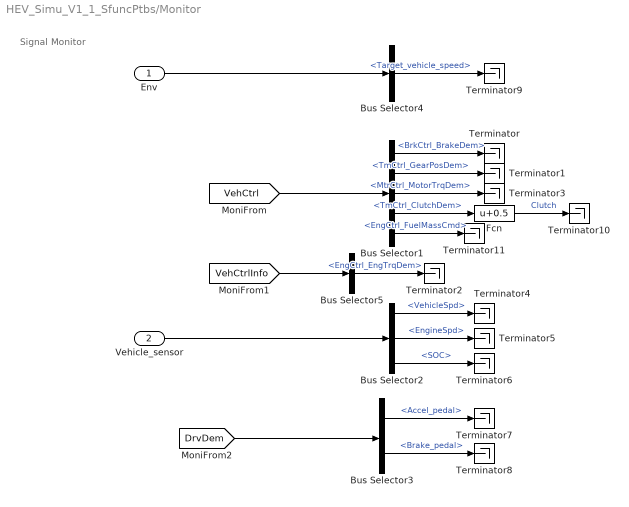
== system HEV_Simu_V1_1_SfuncPtbs/Monitor ==
  note: Signal Monitor
  Env : Inport
  Vehicle_sensor : Inport  Port=2
  Bus Selector1 : BusSelector  OutputSignals=BrakeCtrl.BrkCtrl_BrakeDem,TransmCtrl.TmCtrl_GearPosDem,MotorCtrl.MtrCtrl_MotorTrqDem,TransmCtrl.TmCtrl_ClutchDem,EngineCtrl.EngCtrl_FuelMassCmd
  Bus Selector2 : BusSelector  OutputSignals=Brake_sensor.VehicleSpd,Engine_sensor.EngineSpd,Battery_sensor.SOC
  Bus Selector3 : BusSelector  OutputSignals=Accel_pedal,Brake_pedal
  Bus Selector4 : BusSelector  OutputSignals=Target_vehicle_speed
  Bus Selector5 : BusSelector  OutputSignals=EngineCtrl_Info.EngCtrl_EngTrqDem
  Fcn : Fcn  Expr=u+0.5
  Terminator{,1..11} (12 alike) : Terminator
  wires:
  [VehCtrl] -> Bus Selector1/1
  Vehicle_sensor/1 -> Bus Selector2/1
  Bus Selector1/2 -> Terminator1/1  "<TmCtrl_GearPosDem>"
  Bus Selector1/3 -> Terminator3/1  "<MtrCtrl_MotorTrqDem>"
  Bus Selector2/1 -> Terminator4/1  "<VehicleSpd>"
  Bus Selector2/2 -> Terminator5/1  "<EngineSpd>"
  Bus Selector2/3 -> Terminator6/1  "<SOC>"
  Bus Selector1/1 -> Terminator/1  "<BrkCtrl_BrakeDem>"
  [DrvDem] -> Bus Selector3/1
  Bus Selector3/1 -> Terminator7/1  "<Accel_pedal>"
  Bus Selector3/2 -> Terminator8/1  "<Brake_pedal>"
  Env/1 -> Bus Selector4/1
  Bus Selector4/1 -> Terminator9/1  "<Target_vehicle_speed>"
  [VehCtrlInfo] -> Bus Selector5/1
  Bus Selector5/1 -> Terminator2/1  "<EngCtrl_EngTrqDem>"
  Bus Selector1/4 -> Fcn/1  "<TmCtrl_ClutchDem>"
  Fcn/1 -> Terminator10/1  "Clutch"
  Bus Selector1/5 -> Terminator11/1  "<EngCtrl_FuelMassCmd>"

== system HEV_Simu_V1_1_SfuncPtbs/Controller/Body_Comfort ==
  note: Body Control
  Driver_demand : Inport
  Body_sensor : Inport  Port=2
  Body_Control : Subsystem
  HVAC_Control : Subsystem
  HVAC_Ctrl : Outport
  BodyCtrl : Outport  Port=2
  wires:
  Body_Control/1(BodyCtrl) -> BodyCtrl/1
  Driver_demand/1 -> HVAC_Control/1(Driver_demand), Body_Control/1(Driver_demand)
  Body_sensor/1 -> HVAC_Control/2(Body_sensor), Body_Control/2(Body_sensor)
  HVAC_Control/1(HVAC_Ctrl) -> HVAC_Ctrl/1

== system HEV_Simu_V1_1_SfuncPtbs/Controller/CAN_Variant ==
  note: 1) Add Subsystem or Model blocks as valid variant choices.
      | 2) You cannot connect blocks at this level. At simulation, connectivity is automatically
      | determined, based on the active variant and port name matching.
  Simple_CAN2 : CAN_Lib_V1/Simple_CAN2  SystemSampleTime=-1  VariantControl=VarObj_CanType_Simpl
  Simple_CAN_TW2 : CAN_Lib_V1/Simple_CAN_TW2  SystemSampleTime=-1  VariantControl=VarObj_CanType_Simpl_TW
  VNT_Level1_CAN_TW2 : CAN_Lib_V1/VNT_Level1_CAN_TW2  SystemSampleTime=-1  VariantControl=VarObj_CanType_Simpl_TW
  VNT_Level_2_CAN : CAN_Lib_V1/VNT_Level_2_CAN  SystemSampleTime=-1  VariantControl=VarObj_CanType_VNT_Level_2

== system HEV_Simu_V1_1_SfuncPtbs/Controller/Chassis ==
  note: Chassis Control
  Driver_demand : Inport
  Brake_sensor : Inport  Port=2
  Steer_sensor : Inport  Port=3
  Brake_Control : Subsystem
  Steer_Control : Subsystem
  Brake_ECU_out : Outport
  Steer_ECU_out : Outport  Port=2
  wires:
  Driver_demand/1 -> Brake_Control/1(Driver_demand), Steer_Control/1(Driver_demand)
  Brake_Control/1(BrakeCtrl) -> Brake_ECU_out/1
  Brake_sensor/1 -> Brake_Control/2(Brake_sensor)
  Steer_Control/1(SteerCtrl) -> Steer_ECU_out/1
  Steer_sensor/1 -> Steer_Control/2(Steer_sensor)

== system HEV_Simu_V1_1_SfuncPtbs/Controller/InfoHub ==
  Bus Creator1 : BusCreator  Inputs=2
  VehCtrlInfo : Outport
  wires:
  [HEV_ECU_Info] -> Bus Creator1/1
  [Engine_ECU_Info] -> Bus Creator1/2
  Bus Creator1/1 -> VehCtrlInfo/1  "VehCtrlInfo"

== system HEV_Simu_V1_1_SfuncPtbs/Controller/Infotainment ==
  note: Infotainment
  Driver_demand : Inport
  Env : Inport  Port=2
  Navigation : Subsystem
  Radar_Detection : Subsystem
  wires:
  Env/1 -> Navigation/2(Env), Radar_Detection/2(Env)
  Driver_demand/1 -> Radar_Detection/1(Driver_demand), Navigation/1(Driver_demand)

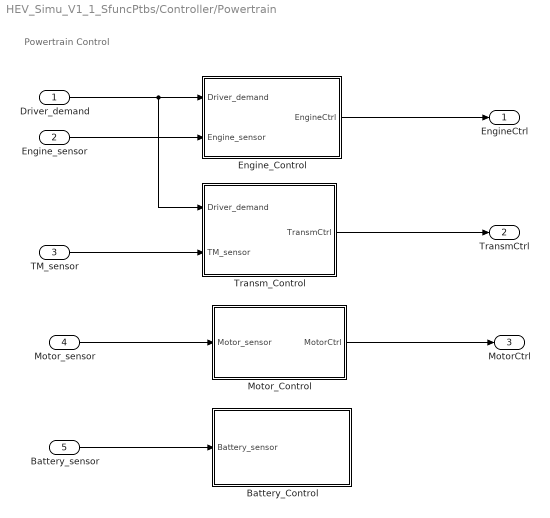
== system HEV_Simu_V1_1_SfuncPtbs/Controller/Powertrain ==
  note: Powertrain Control
  Driver_demand : Inport
  Engine_sensor : Inport  Port=2
  TM_sensor : Inport  Port=3
  Motor_sensor : Inport  Port=4
  Battery_sensor : Inport  Port=5
  Battery_Control : Subsystem
  Engine_Control : Subsystem
  Motor_Control : Subsystem
  Transm_Control : Subsystem
  EngineCtrl : Outport
  TransmCtrl : Outport  Port=2
  MotorCtrl : Outport  Port=3
  wires:
  Driver_demand/1 -> Transm_Control/1(Driver_demand), Engine_Control/1(Driver_demand)
  Motor_Control/1(MotorCtrl) -> MotorCtrl/1
  Motor_sensor/1 -> Motor_Control/1(Motor_sensor)
  Battery_sensor/1 -> Battery_Control/1(Battery_sensor)
  Engine_Control/1(EngineCtrl) -> EngineCtrl/1
  Engine_sensor/1 -> Engine_Control/2(Engine_sensor)
  Transm_Control/1(TransmCtrl) -> TransmCtrl/1
  TM_sensor/1 -> Transm_Control/2(TM_sensor)

== system HEV_Simu_V1_1_SfuncPtbs/Controller/Vehicle ==
  note: Vehicle Integrated Control
  Driver_demand : Inport
  Env : Inport  Port=2
  HEV_sensor : Inport  Port=3
  HEV_Control : Subsystem
  Vehicle_Motion_Control : Subsystem
  wires:
  Env/1 -> Vehicle_Motion_Control/1(Env)
  Driver_demand/1 -> HEV_Control/1(Driver_demand)
  HEV_sensor/1 -> HEV_Control/2(HEV_sensor)

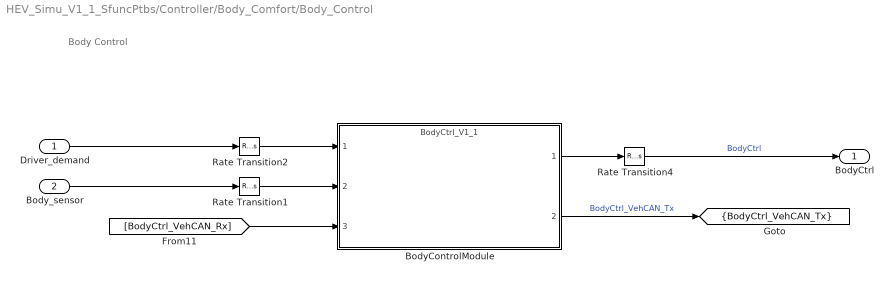
== system HEV_Simu_V1_1_SfuncPtbs/Controller/Body_Comfort/Body_Control ==
  note: Body Control
  Driver_demand : Inport
  Body_sensor : Inport  Port=2
  BodyControlModule : ModelReference  ModelNameDialog=BodyCtrl_V1_1.slx  SimulationMode=Normal  ModelReferenceVersion=0.1.18
  Rate Transition1 : RateTransition  Deterministic=off
      settings: AttributesFormatString=<Deterministic=%<Deterministic>>
  Rate Transition2 : RateTransition  Deterministic=off
      settings: AttributesFormatString=<Deterministic=%<Deterministic>>
  Rate Transition4 : RateTransition  Deterministic=off
      settings: AttributesFormatString=<Deterministic=%<Deterministic>>
  BodyCtrl : Outport
  tag scope: BodyCtrl_VehCAN_Tx=scoped
  wires:
  Driver_demand/1 -> Rate Transition2/1
  Rate Transition2/1 -> BodyControlModule/1
  BodyControlModule/1 -> Rate Transition4/1
  [BodyCtrl_VehCAN_Rx] -> BodyControlModule/3
  BodyControlModule/2 -> [BodyCtrl_VehCAN_Tx]  "BodyCtrl_VehCAN_Tx"
  Rate Transition4/1 -> BodyCtrl/1  "BodyCtrl"
  Body_sensor/1 -> Rate Transition1/1
  Rate Transition1/1 -> BodyControlModule/2

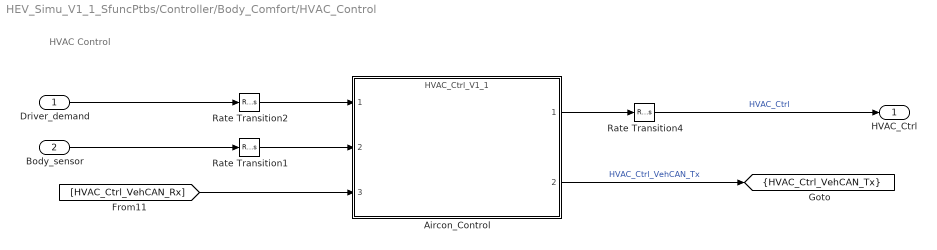
== system HEV_Simu_V1_1_SfuncPtbs/Controller/Body_Comfort/HVAC_Control ==
  note: HVAC Control
  Driver_demand : Inport
  Body_sensor : Inport  Port=2
  Aircon_Control : ModelReference  ModelNameDialog=HVAC_Ctrl_V1_1.slx  SimulationMode=Normal  ModelReferenceVersion=0.1.27
  Rate Transition1 : RateTransition  Deterministic=off
      settings: AttributesFormatString=<Deterministic=%<Deterministic>>
  Rate Transition2 : RateTransition  Deterministic=off
      settings: AttributesFormatString=<Deterministic=%<Deterministic>>
  Rate Transition4 : RateTransition  Deterministic=off
      settings: AttributesFormatString=<Deterministic=%<Deterministic>>
  HVAC_Ctrl : Outport
  tag scope: HVAC_Ctrl_VehCAN_Tx=scoped
  wires:
  Rate Transition1/1 -> Aircon_Control/2
  Body_sensor/1 -> Rate Transition1/1
  Rate Transition4/1 -> HVAC_Ctrl/1  "HVAC_Ctrl"
  Aircon_Control/2 -> [HVAC_Ctrl_VehCAN_Tx]  "HVAC_Ctrl_VehCAN_Tx"
  [HVAC_Ctrl_VehCAN_Rx] -> Aircon_Control/3
  Aircon_Control/1 -> Rate Transition4/1
  Rate Transition2/1 -> Aircon_Control/1
  Driver_demand/1 -> Rate Transition2/1

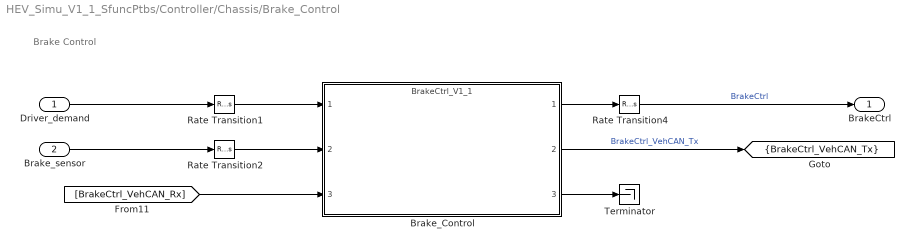
== system HEV_Simu_V1_1_SfuncPtbs/Controller/Chassis/Brake_Control ==
  note: Brake Control
  Driver_demand : Inport
  Brake_sensor : Inport  Port=2
  Brake_Control : ModelReference  ModelNameDialog=BrakeCtrl_V1_1.slx  SimulationMode=Normal  ModelReferenceVersion=1.0.25
  Rate Transition1 : RateTransition  Deterministic=off
      settings: AttributesFormatString=<Deterministic=%<Deterministic>>
  Rate Transition2 : RateTransition  Deterministic=off
      settings: AttributesFormatString=<Deterministic=%<Deterministic>>
  Rate Transition4 : RateTransition  Deterministic=off
      settings: AttributesFormatString=<Deterministic=%<Deterministic>>
  Terminator : Terminator
  BrakeCtrl : Outport
  tag scope: BrakeCtrl_VehCAN_Tx=scoped
  wires:
  Rate Transition2/1 -> Brake_Control/2
  Driver_demand/1 -> Rate Transition1/1
  Rate Transition1/1 -> Brake_Control/1
  Brake_sensor/1 -> Rate Transition2/1
  Brake_Control/3 -> Terminator/1
  [BrakeCtrl_VehCAN_Rx] -> Brake_Control/3
  Rate Transition4/1 -> BrakeCtrl/1  "BrakeCtrl"
  Brake_Control/1 -> Rate Transition4/1
  Brake_Control/2 -> [BrakeCtrl_VehCAN_Tx]  "BrakeCtrl_VehCAN_Tx"

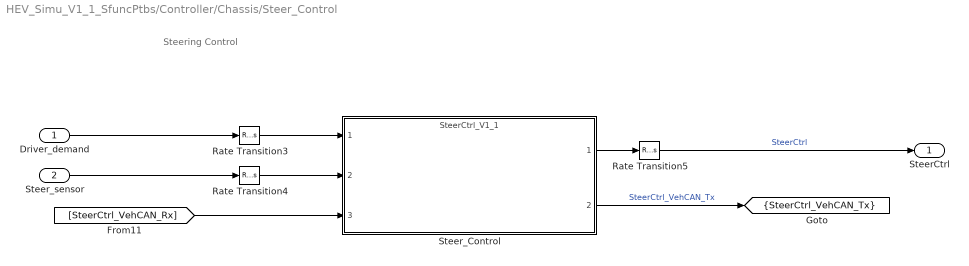
== system HEV_Simu_V1_1_SfuncPtbs/Controller/Chassis/Steer_Control ==
  note: Steering Control
  Driver_demand : Inport
  Steer_sensor : Inport  Port=2
  Rate Transition3 : RateTransition  Deterministic=off
      settings: AttributesFormatString=<Deterministic=%<Deterministic>>
  Rate Transition4 : RateTransition  Deterministic=off
      settings: AttributesFormatString=<Deterministic=%<Deterministic>>
  Rate Transition5 : RateTransition  Deterministic=off
      settings: AttributesFormatString=<Deterministic=%<Deterministic>>
  Steer_Control : ModelReference  ModelNameDialog=SteerCtrl_V1_1.slx  SimulationMode=Normal  ModelReferenceVersion=0.1.18
  SteerCtrl : Outport
  tag scope: SteerCtrl_VehCAN_Tx=scoped
  wires:
  Rate Transition4/1 -> Steer_Control/2
  Driver_demand/1 -> Rate Transition3/1
  Steer_Control/1 -> Rate Transition5/1
  Steer_sensor/1 -> Rate Transition4/1
  [SteerCtrl_VehCAN_Rx] -> Steer_Control/3
  Rate Transition3/1 -> Steer_Control/1
  Rate Transition5/1 -> SteerCtrl/1  "SteerCtrl"
  Steer_Control/2 -> [SteerCtrl_VehCAN_Tx]  "SteerCtrl_VehCAN_Tx"

== system HEV_Simu_V1_1_SfuncPtbs/Controller/Infotainment/Navigation ==
  note: Navigation
  Driver_demand : Inport
  Env : Inport  Port=2
  NAVI : ModelReference  ModelNameDialog=NAVI_V1_1.slx  SimulationMode=Normal  ModelReferenceVersion=0.1.19
  Rate Transition1 : RateTransition  Deterministic=off
      settings: AttributesFormatString=<Deterministic=%<Deterministic>>
  Rate Transition4 : RateTransition  Deterministic=off
      settings: AttributesFormatString=<Deterministic=%<Deterministic>>
  tag scope: NAVI_InfoCAN_Tx=scoped
  wires:
  Rate Transition1/1 -> NAVI/1
  Driver_demand/1 -> Rate Transition1/1
  [NAVI_InfoCAN_Rx] -> NAVI/3
  NAVI/1 -> [NAVI_InfoCAN_Tx]  "NAVI_InfoCAN_Tx"
  Env/1 -> Rate Transition4/1
  Rate Transition4/1 -> NAVI/2

== system HEV_Simu_V1_1_SfuncPtbs/Controller/Infotainment/Radar_Detection ==
  note: Radar Detection
  Driver_demand : Inport
  Env : Inport  Port=2
  Radar_Detection : ModelReference  ModelNameDialog=Radar_V1_1.slx  SimulationMode=Normal  ModelReferenceVersion=0.1.19
  Rate Transition1 : RateTransition  Deterministic=off
      settings: AttributesFormatString=<Deterministic=%<Deterministic>>
  Rate Transition4 : RateTransition  Deterministic=off
      settings: AttributesFormatString=<Deterministic=%<Deterministic>>
  tag scope: Radar_InfoCAN_Tx=scoped
  wires:
  Rate Transition1/1 -> Radar_Detection/2
  Env/1 -> Rate Transition1/1
  [Radar_InfoCAN_Rx] -> Radar_Detection/3
  Radar_Detection/1 -> [Radar_InfoCAN_Tx]  "Radar_InfoCAN_Tx"
  Driver_demand/1 -> Rate Transition4/1
  Rate Transition4/1 -> Radar_Detection/1

== system HEV_Simu_V1_1_SfuncPtbs/Controller/Powertrain/Battery_Control ==
  note: Battery Control
  Battery_sensor : Inport
  Battery_Control : ModelReference  ModelNameDialog=BatteryCtrl_V1_1.slx  SimulationMode=Normal  ModelReferenceVersion=0.1.24
  Rate Transition1 : RateTransition  Deterministic=off
      settings: AttributesFormatString=<Deterministic=%<Deterministic>>
  tag scope: BatteryCtrl_PwtrCAN_Tx=scoped
  wires:
  Battery_sensor/1 -> Rate Transition1/1
  [BatteryCtrl_PwtrCAN_Rx] -> Battery_Control/2
  Rate Transition1/1 -> Battery_Control/1
  Battery_Control/1 -> [BatteryCtrl_PwtrCAN_Tx]  "BatteryCtrl_PwtrCAN_Tx"

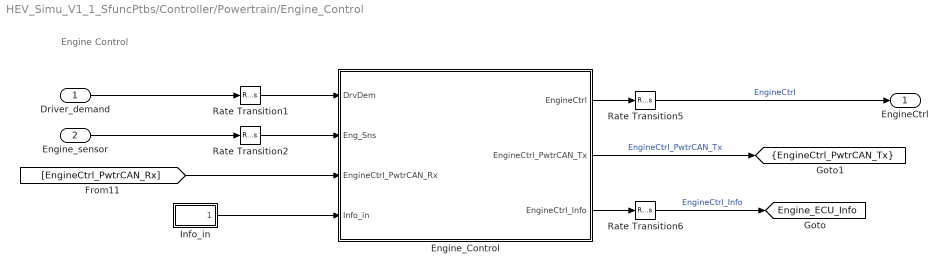
== system HEV_Simu_V1_1_SfuncPtbs/Controller/Powertrain/Engine_Control ==
  note: Engine Control
  Driver_demand : Inport
  Engine_sensor : Inport  Port=2
  Engine_Control : Subsystem  Variant=on
  Info_in : Subsystem
  Rate Transition{1..2,5..6} (4 alike) : RateTransition  Deterministic=off
      settings: AttributesFormatString=<Deterministic=%<Deterministic>>
  EngineCtrl : Outport
  tag scope: EngineCtrl_PwtrCAN_Tx=scoped, Engine_ECU_Info=global
  wires:
  Driver_demand/1 -> Rate Transition1/1
  Engine_sensor/1 -> Rate Transition2/1
  Rate Transition5/1 -> EngineCtrl/1  "EngineCtrl"
  Rate Transition6/1 -> [Engine_ECU_Info]  "EngineCtrl_Info"
  Engine_Control/2(" EngineCtrl_PwtrCAN_Tx") -> [EngineCtrl_PwtrCAN_Tx]  "EngineCtrl_PwtrCAN_Tx"
  Rate Transition1/1 -> Engine_Control/1("DrvDem ")
  Rate Transition2/1 -> Engine_Control/2("Eng_Sns ")
  [EngineCtrl_PwtrCAN_Rx] -> Engine_Control/3(EngineCtrl_PwtrCAN_Rx)
  Info_in/1(Info_in) -> Engine_Control/4("Info_in ")
  Engine_Control/1(" EngineCtrl") -> Rate Transition5/1
  Engine_Control/3(" EngineCtrl_Info") -> Rate Transition6/1

== system HEV_Simu_V1_1_SfuncPtbs/Controller/Powertrain/Motor_Control ==
  note: Motor Control
  Motor_sensor : Inport
  Motor_Control : ModelReference  ModelNameDialog=MotorCtrl_V1_1.slx  SimulationMode=Normal  ModelReferenceVersion=1.0.23
  Rate Transition1 : RateTransition  Deterministic=off
      settings: AttributesFormatString=<Deterministic=%<Deterministic>>
  Rate Transition3 : RateTransition  Deterministic=off
      settings: AttributesFormatString=<Deterministic=%<Deterministic>>
  Terminator : Terminator
  MotorCtrl : Outport
  tag scope: MotorCtrl_PwtrCAN_Tx=scoped
  wires:
  Rate Transition1/1 -> Motor_Control/1
  [MotorCtrl_PwtrCAN_Rx] -> Motor_Control/2
  Motor_sensor/1 -> Rate Transition1/1
  Motor_Control/3 -> Terminator/1
  Rate Transition3/1 -> MotorCtrl/1  "MotorCtrl"
  Motor_Control/1 -> Rate Transition3/1
  Motor_Control/2 -> [MotorCtrl_PwtrCAN_Tx]  "MotorCtrl_PwtrCAN_Tx"

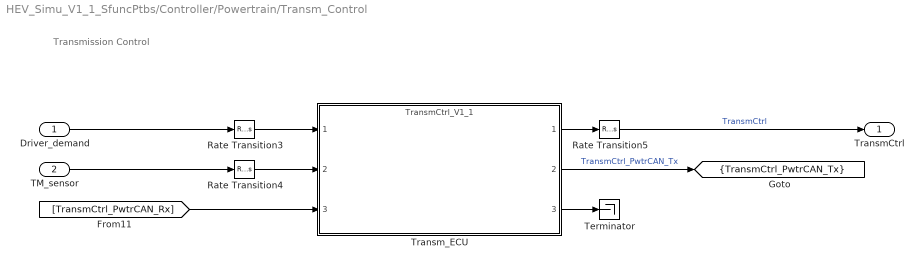
== system HEV_Simu_V1_1_SfuncPtbs/Controller/Powertrain/Transm_Control ==
  note: Transmission Control
  Driver_demand : Inport
  TM_sensor : Inport  Port=2
  Rate Transition3 : RateTransition  Deterministic=off
      settings: AttributesFormatString=<Deterministic=%<Deterministic>>
  Rate Transition4 : RateTransition  Deterministic=off
      settings: AttributesFormatString=<Deterministic=%<Deterministic>>
  Rate Transition5 : RateTransition  Deterministic=off
      settings: AttributesFormatString=<Deterministic=%<Deterministic>>
  Terminator : Terminator
  Transm_ECU : ModelReference  ModelNameDialog=TransmCtrl_V1_1.slx  SimulationMode=Normal  ModelReferenceVersion=1.0.43
  TransmCtrl : Outport
  tag scope: TransmCtrl_PwtrCAN_Tx=scoped
  wires:
  Rate Transition4/1 -> Transm_ECU/2
  Transm_ECU/3 -> Terminator/1
  Driver_demand/1 -> Rate Transition3/1
  TM_sensor/1 -> Rate Transition4/1
  [TransmCtrl_PwtrCAN_Rx] -> Transm_ECU/3
  Rate Transition3/1 -> Transm_ECU/1
  Rate Transition5/1 -> TransmCtrl/1  "TransmCtrl"
  Transm_ECU/1 -> Rate Transition5/1
  Transm_ECU/2 -> [TransmCtrl_PwtrCAN_Tx]  "TransmCtrl_PwtrCAN_Tx"

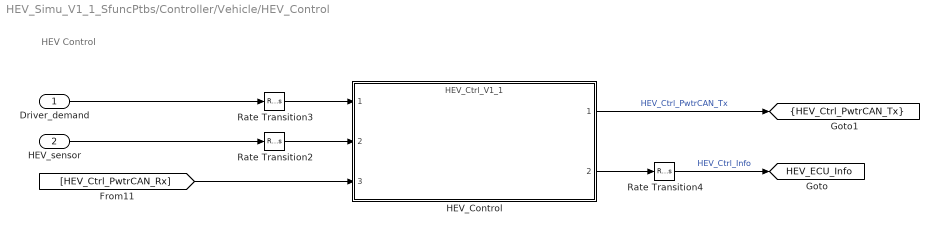
== system HEV_Simu_V1_1_SfuncPtbs/Controller/Vehicle/HEV_Control ==
  note: HEV Control
  Driver_demand : Inport
  HEV_sensor : Inport  Port=2
  HEV_Control : ModelReference  ModelNameDialog=HEV_Ctrl_V1_1.slx  SimulationMode=Normal  ModelReferenceVersion=1.0.62
  Rate Transition2 : RateTransition  Deterministic=off
      settings: AttributesFormatString=<Deterministic=%<Deterministic>>
  Rate Transition3 : RateTransition  Deterministic=off
      settings: AttributesFormatString=<Deterministic=%<Deterministic>>
  Rate Transition4 : RateTransition  Deterministic=off
      settings: AttributesFormatString=<Deterministic=%<Deterministic>>
  tag scope: HEV_Ctrl_PwtrCAN_Tx=scoped, HEV_ECU_Info=global
  wires:
  Driver_demand/1 -> Rate Transition3/1
  [HEV_Ctrl_PwtrCAN_Rx] -> HEV_Control/3
  HEV_sensor/1 -> Rate Transition2/1
  Rate Transition2/1 -> HEV_Control/2
  HEV_Control/2 -> Rate Transition4/1
  Rate Transition4/1 -> [HEV_ECU_Info]  "HEV_Ctrl_Info"
  HEV_Control/1 -> [HEV_Ctrl_PwtrCAN_Tx]  "HEV_Ctrl_PwtrCAN_Tx"
  Rate Transition3/1 -> HEV_Control/1

== system HEV_Simu_V1_1_SfuncPtbs/Controller/Vehicle/Vehicle_Motion_Control ==
  note: Vehicle Motion Control
  Env : Inport
  Rate Transition1 : RateTransition  Deterministic=off
      settings: AttributesFormatString=<Deterministic=%<Deterministic>>
  Vehicle_Motion_Control : ModelReference  ModelNameDialog=VM_Ctrl_V1_1.slx  SimulationMode=Normal  ModelReferenceVersion=0.1.28
  tag scope: VM_Ctrl_VehCAN_Tx=scoped
  wires:
  Vehicle_Motion_Control/1 -> [VM_Ctrl_VehCAN_Tx]  "VM_Ctrl_VehCAN_Tx"
  Rate Transition1/1 -> Vehicle_Motion_Control/1
  Env/1 -> Rate Transition1/1
  [VM_Ctrl_VehCAN_Rx] -> Vehicle_Motion_Control/2

== system HEV_Simu_V1_1_SfuncPtbs/Controller/Powertrain/Engine_Control/Engine_Control ==
  "DrvDem " : Inport
  "Eng_Sns " : Inport  Port=2
  EngineCtrl_PwtrCAN_Rx : Inport  Port=3
  "Info_in " : Inport  Port=4
  EngineCtrl_V1.slx : ModelReference  ModelNameDialog=EngineCtrl_V1_1.slx  SimulationMode=Normal  VariantControl=VarObj_EngEcu_Simple  ModelReferenceVersion=1.0.27
  EngineCtrl_V2.slx : ModelReference  ModelNameDialog=EngineCtrl_V2.slx  SimulationMode=Normal  VariantControl=VarObj_EngEcu_Medium  ModelReferenceVersion=1.0.8
  " EngineCtrl" : Outport
  " EngineCtrl_PwtrCAN_Tx" : Outport  Port=2
  " EngineCtrl_Info" : Outport  Port=3

== system HEV_Simu_V1_1_SfuncPtbs/Controller/Powertrain/Engine_Control/Info_in ==
  Bus Creator1 : BusCreator  Inputs=1
  Constant : Constant
  Info_in : Outport
  wires:
  Constant/1 -> Bus Creator1/1  "dummy"
  Bus Creator1/1 -> Info_in/1  "Info_in"
